simulink model "YY2"  (R2015a)
settings: Solver=ode45  StartTime=0.0  StopTime=10.0  RelTol=1e-3
libraries: powerlib x12
settings Model: Creator=ASUS  LastModifiedBy=ASUS

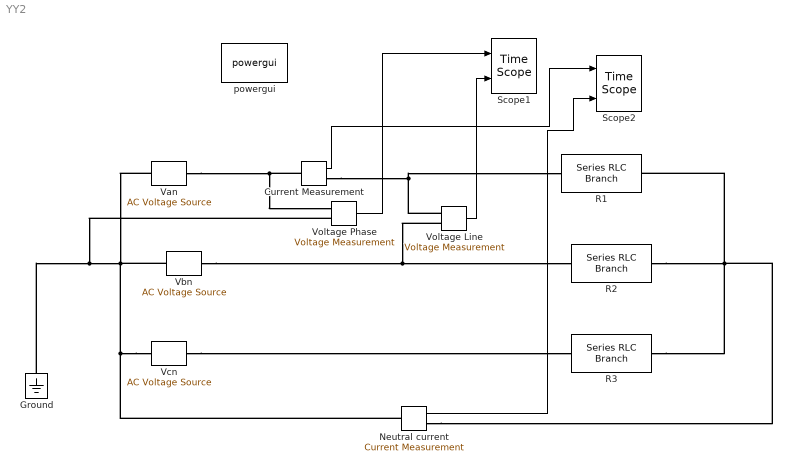
== system YY2 ==
  Current Measurement : powerlib/Measurements/Current Measurement  PhasorSimulation=off  OutputType=Complex  PSBequivalent=0
  Ground : powerlib/Elements/Ground  LConnTagsString=a
  Neutral current : powerlib/Measurements/Current Measurement  PhasorSimulation=off  OutputType=Complex  PSBequivalent=0
  R1 : powerlib/Elements/Series RLC Branch  LConnTagsString=__new0  RConnTagsString=__new0  BranchType=R  Resistance=100  Inductance=1e-3  SetiL0=off  InitialCurrent=0  Capacitance=1e-6  Setx0=off  InitialVoltage=0  Measurements=None
  R2 : powerlib/Elements/Series RLC Branch  LConnTagsString=__new0  RConnTagsString=__new0  BranchType=R  Resistance=100  Inductance=1e-3  SetiL0=off  InitialCurrent=0  Capacitance=1e-6  Setx0=off  InitialVoltage=0  Measurements=None
  R3 : powerlib/Elements/Series RLC Branch  LConnTagsString=__new0  RConnTagsString=__new0  BranchType=R  Resistance=100  Inductance=1e-3  SetiL0=off  InitialCurrent=0  Capacitance=1e-6  Setx0=off  InitialVoltage=0  Measurements=None
  Scope1 : TimeScope  NumInputPorts=2
  Scope2 : TimeScope  NumInputPorts=2
  Van : powerlib/Electrical Sources/AC Voltage Source  Amplitude=220*1.4142  Phase=0  Frequency=50  SampleTime=0  Measurements=None
  Vbn : powerlib/Electrical Sources/AC Voltage Source  Amplitude=220*1.4142  Phase=-120  Frequency=50  SampleTime=0  Measurements=None
  Vcn : powerlib/Electrical Sources/AC Voltage Source  Amplitude=220*1.4142  Phase=120  Frequency=50  SampleTime=0  Measurements=None
  Voltage Line : powerlib/Measurements/Voltage Measurement  PhasorSimulation=off  OutputType=Complex  PSBequivalent=0
  Voltage Phase : powerlib/Measurements/Voltage Measurement  PhasorSimulation=off  OutputType=Complex  PSBequivalent=0
  powergui : powerlib/powergui  Priority=1  SimulationMode=Continuous  SolverType=Tustin/Backward Euler (TBE)  SampleTime=50e-6  frequency=60  SPID=off  DisableSnubberDevices=off  DisableRonSwitches=off  DisableVfSwitches=off  SwTol=0  DisplayEquations=off  Interpol=off  methode=off  Ts=100  FunctionMessages=off  echomessages=off  HookPort=off  EnableUseOfTLC=off  x0status=blocks  frequencyindice=50  Pbase=100e6  ErrMax=1e-4  Iterations=50  UnitsV=kV  UnitsW=MW  buscounter=0  RestoreLinks=warning  ResistiveCurrentMeasurement=off  Frange=[0:2:500]  Ylog=off  Xlog=on  ShowGrid=off  save=off  variable=ZData  structure=0  ZoomFFT=off  StartTime=0.0  cycles=1  DisplayStyle=1  fundamental=60  FreqAxis=off  MaxFrequency=1000  frequencyindicesteady=1  RmsSteady=1  display=off
  wires:
  Voltage Phase/1 -> Scope1/1
  Voltage Line/1 -> Scope1/2
  Current Measurement/1 -> Scope2/1
  Neutral current/1 -> Scope2/2
  connections:
  Vcn/LConn1 -- Van/LConn1 -- Vbn/LConn1 -- Voltage Phase/LConn2 -- Ground/LConn1 -- Neutral current/LConn1
  R2/RConn1 -- Neutral current/RConn1 -- R1/RConn1 -- R3/RConn1
  Vbn/RConn1 -- R2/LConn1 -- Voltage Line/LConn2
  Voltage Line/LConn1 -- R1/LConn1 -- Current Measurement/RConn1
  Van/RConn1 -- Voltage Phase/LConn1 -- Current Measurement/LConn1
  Vcn/RConn1 -- R3/LConn1
